simulink model "Example_Hydraulic_ValveThermostatic"  (R2013b)
settings: Solver=ode45  StartTime=0.0  StopTime=600  RelTol=1e-3
libraries: carnot x8, simulink x1
settings Model: Creator=drhf  LastModifiedBy=drhf
settings DataIOCC: SignalLoggingSaveFormat=ModelDataLogs
settings OptimizationCC: ExpressionDepthLimit=2147483647
settings DebuggingCC: FcnCallInpInsideContextMsg=EnableAllAsWarning  StateNameClashWarn=warning
settings GRTTargetCC: CombineOutputUpdateFcns=off  GRTInterface=on

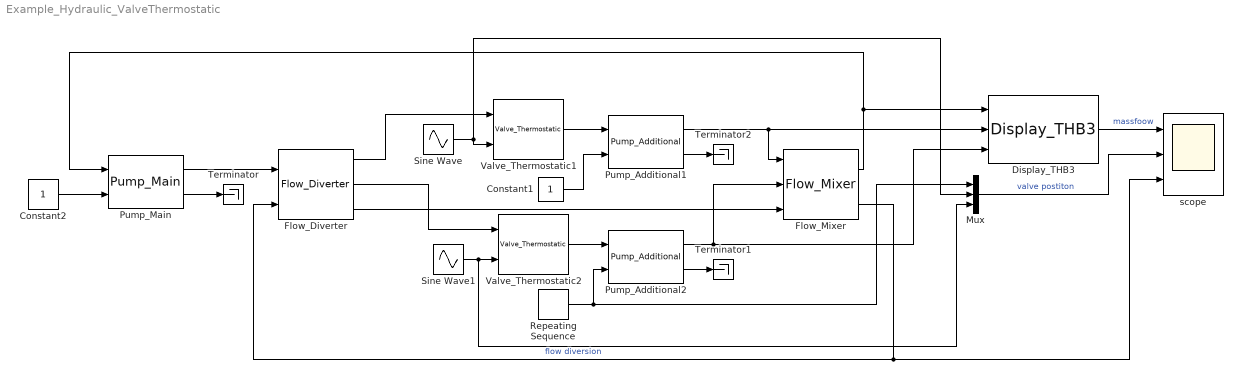
== system Example_Hydraulic_ValveThermostatic ==
  Constant1 : Constant
  Constant2 : Constant
  Display_THB3 : carnot/Outputs/Display_THB3  t=off  m=on  p=off  id=off  mix=off  d=off
  Flow_Diverter : carnot/Hydraulics/Flow_Diverter
  Flow_Mixer : carnot/Hydraulics/Flow_Mixer  t=1
  Mux : Mux  Inputs=3
  Pump_Additional1 : carnot/Hydraulics/Pump_Additional  a0=2.0e4  a1=-7000  a2=0 %-3e-3  dia=0.025  t1=1  ua=0  mcp=0  tamb=0
  Pump_Additional2 : carnot/Hydraulics/Pump_Additional  a0=2.0e4  a1=-7000  a2=0 %-3e-3  dia=0.025  t1=1  ua=0  mcp=0  tamb=0
  Pump_Main : carnot/Hydraulics/Pump_Main  a0=2.7e4  a1=-1.2e4  a2=0%-3e-3  dia=0.025  t1=1  p0=3e5  IDchk=off  fluid_id=Water  mix=0  ua=1  mcp=500  tamb=20
  Repeating Sequence : simulink/Sources/Repeating Sequence  rep_seq_t=[0 10 20 500]  rep_seq_y=[0 0 1 1]
  Sine Wave : Sin  Amplitude=4  Bias=20  Frequency=1/60  SampleTime=0
  Sine Wave1 : Sin  Amplitude=4  Bias=20  Frequency=1/60  Phase=pi  SampleTime=0
  Terminator : Terminator
  Terminator1 : Terminator
  Terminator2 : Terminator
  Valve_Thermostatic1 : carnot/Hydraulics/Valve_Thermostatic  Tset=20  prange=3  op=0.5  bl=0.1  ts=1  dia=0.02  vpos=[0 0.1 1]  vqua=[1e6 1e6 1]
  Valve_Thermostatic2 : carnot/Hydraulics/Valve_Thermostatic  Tset=20  prange=3  op=0.5  bl=0.1  ts=1  dia=0.02  vpos=[0 0.1 1]  vqua=[1e6 1e6 1]
  scope : Scope  NumInputPorts=3
      settings: TickLabels=on  YMin=0~-5~-5  YMax=5~5~5
  wires:
  Constant2/1 -> Pump_Main/2
  Pump_Main/2 -> Terminator/1
  Sine Wave/1 -> Mux/2, Valve_Thermostatic1/2
  Pump_Main/1 -> Flow_Diverter/1
  Flow_Diverter/1 -> Valve_Thermostatic1/1
  Sine Wave1/1 -> Mux/3, Valve_Thermostatic2/2
  Flow_Diverter/2 -> Valve_Thermostatic2/1
  Flow_Diverter/3 -> Flow_Mixer/3
  Flow_Mixer/2 -> scope/3, Flow_Diverter/2  "flow diversion"
  Flow_Mixer/1 -> Pump_Main/1, Display_THB3/1
  Display_THB3/1 -> scope/1  "massfoow"
  Mux/1 -> scope/2  "valve postiton"
  Valve_Thermostatic2/1 -> Pump_Additional2/1
  Pump_Additional2/1 -> Flow_Mixer/2, Display_THB3/3
  Pump_Additional2/2 -> Terminator1/1
  Repeating Sequence/1 -> Mux/1, Pump_Additional2/2
  Valve_Thermostatic1/1 -> Pump_Additional1/1
  Constant1/1 -> Pump_Additional1/2
  Pump_Additional1/1 -> Flow_Mixer/1, Display_THB3/2
  Pump_Additional1/2 -> Terminator2/1
